simulink model "FSMK_DRC"  (R2016b)
settings: Solver=ode5  StartTime=0.0  StopTime=800  FixedStep=1  RelTol=1e-3  EnableMultiTasking=on
libraries: fuzblock x1
settings Model: Creator=p4wp4w  LastModifiedBy=ABLAH
settings DataIOCC: LimitDataPoints=on  SaveFormat=Array
settings OptimizationCC: LifeSpan=inf
settings DebuggingCC: SFUnexpectedBacktrackingDiag=warning  SFNoUnconditionalDefaultTransitionDiag=warning  SFExecutionAtInitializationDiag=none
settings HardwareCC: ProdBitPerPointer=32  ProdBitPerSizeT=32  ProdBitPerPtrDiffT=32  ProdLargestAtomicFloat=None  ProdIntDivRoundTo=Undefined  ProdEndianess=Unspecified  ProdWordSize=32  ProdHWDeviceType=32-bit Generic
settings ModelReferenceCC: PropagateSignalLabelsOutOfModel=off
settings GRTTargetCC: TargetLangStandard=C89/C90 (ANSI)  GeneratePreprocessorConditionals=Disable all
settings ConfigComp: CovMetricSettings=dw  CovHtmlReporting=on  CovSaveCumulativeToWorkspaceVar=on  CovSaveSingleToWorkspaceVar=on  CovExternalEMLEnable=off

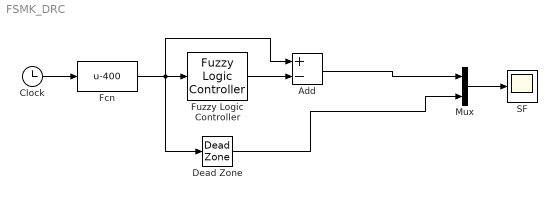
== system FSMK_DRC ==
  Add : Sum  Inputs=+-
  Clock : Clock
  Dead Zone : DeadZone  LowerValue=-180  UpperValue=180  SaturateOnIntegerOverflow=on
  Fcn : Fcn  Expr=u-400
  Fuzzy Logic Controller : fuzblock/Fuzzy Logic  Controller  fis='FSMO.fis'
  Mux : Mux  Inputs=2
  SF : Scope
  wires:
  Clock/1 -> Fcn/1
  Fcn/1 -> Dead Zone/1, Add/1, Fuzzy Logic Controller/1
  Fuzzy Logic Controller/1 -> Add/2
  Dead Zone/1 -> Mux/2
  Mux/1 -> SF/1
  Add/1 -> Mux/1
